simulink model "Tempreture_Heating_System"  (R2024a)
settings: Solver=VariableStepAuto  StartTime=0.0  StopTime=3000  RelTol=1e-3
values from neighbouring files (symbols this model uses):
  efficiency = 0.98    [Inputs.m]
settings Model: Creator=DELL  LastModifiedBy=DELL

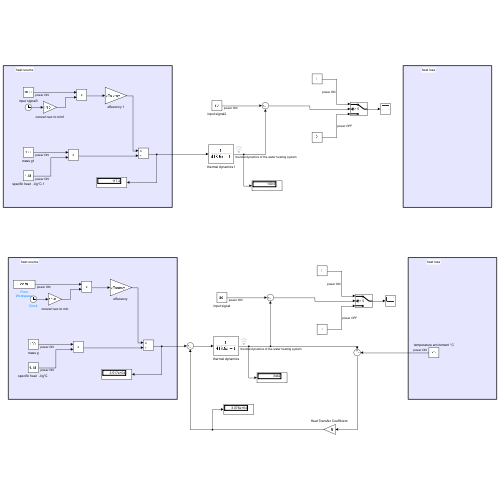
[thumbnail: Simulink's stored preview of the top-level diagram]
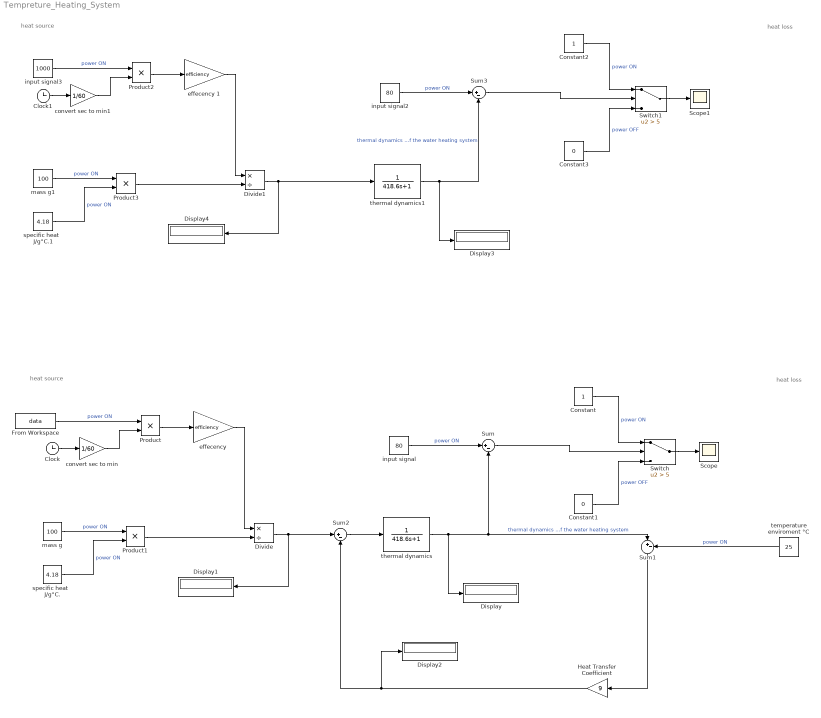
== system Tempreture_Heating_System ==
  note: heat loss
  note: heat source
  note: heat source
  note: heat loss
  Clock : Clock
  Clock1 : Clock
  Constant : Constant
  Constant1 : Constant  Value=0
  Constant2 : Constant
  Constant3 : Constant  Value=0
  Display{,1..4} (5 alike) : Display
  Divide : Product  Inputs=*/
  Divide1 : Product  Inputs=*/
  From Workspace : FromWorkspace  VariableName=data  SampleTime=-1
  "Heat Transfer Coefficient " : Gain  Gain=9
  Product{,1..3} (4 alike) : Product
  Scope : Scope
  Scope1 : Scope
  Sum{,1..3} (4 alike) : Sum  Inputs=|+-
  Switch : Switch  Criteria=u2 > Threshold  Threshold=5  SaturateOnIntegerOverflow=off  InputSameDT=off
  Switch1 : Switch  Criteria=u2 > Threshold  Threshold=5  SaturateOnIntegerOverflow=off  InputSameDT=off
  convert sec to min : Gain  Gain=1/60
  convert sec to min1 : Gain  Gain=1/60
  "effecency " : Gain  Gain=efficiency
  effecency 1 : Gain  Gain=efficiency
  input signal : Constant  Value=80
  input signal2 : Constant  Value=80
  input signal3 : Constant  Value=1000
  mass g : Constant  Value=100
  mass g1 : Constant  Value=100
  specific heat   J/g°C. : Constant  Value=4.18
  specific heat   J/g°C.1 : Constant  Value=4.18
  temperature enviroment °C : Constant  Value=25
  thermal dynamics : TransferFcn  Numerator=1  Denominator=[418.6 1]
  thermal dynamics1 : TransferFcn  Numerator=1  Denominator=[418.6 1]
  wires:
  thermal dynamics/1 -> Display/1, Sum/2, Sum1/1  "thermal dynamics of the water heating system"
  Constant/1 -> Switch/1  "power ON"
  Constant1/1 -> Switch/3  "power OFF"
  Switch/1 -> Scope/1
  Product/1 -> "effecency "/1
  "effecency "/1 -> Divide/1
  mass g/1 -> Product1/1  "power ON"
  specific heat   J/g°C./1 -> Product1/2  "power ON"
  Product1/1 -> Divide/2
  Clock/1 -> convert sec to min/1
  convert sec to min/1 -> Product/2
  Divide/1 -> Sum2/1, Display1/1
  input signal/1 -> Sum/1  "power ON"
  Sum/1 -> Switch/2
  temperature enviroment °C/1 -> Sum1/2  "power ON"
  Sum1/1 -> "Heat Transfer Coefficient "/1
  "Heat Transfer Coefficient "/1 -> Display2/1, Sum2/2
  Sum2/1 -> thermal dynamics/1
  From Workspace/1 -> Product/1  "power ON"
  Clock1/1 -> convert sec to min1/1
  Product2/1 -> effecency 1/1
  effecency 1/1 -> Divide1/1
  mass g1/1 -> Product3/1  "power ON"
  specific heat   J/g°C.1/1 -> Product3/2  "power ON"
  input signal2/1 -> Sum3/1  "power ON"
  Sum3/1 -> Switch1/2
  Product3/1 -> Divide1/2
  convert sec to min1/1 -> Product2/2
  Switch1/1 -> Scope1/1
  Divide1/1 -> thermal dynamics1/1, Display4/1
  thermal dynamics1/1 -> Display3/1, Sum3/2  "thermal dynamics of the water heating system"
  Constant3/1 -> Switch1/3  "power OFF"
  Constant2/1 -> Switch1/1  "power ON"
  input signal3/1 -> Product2/1  "power ON"
